simulink model "gerbang_logika"  (R2025a)
settings: Solver=VariableStepAuto  StartTime=0.0  StopTime=10.0  RelTol=1e-3
settings Model: Creator=pasha  LastModifiedBy=pasha

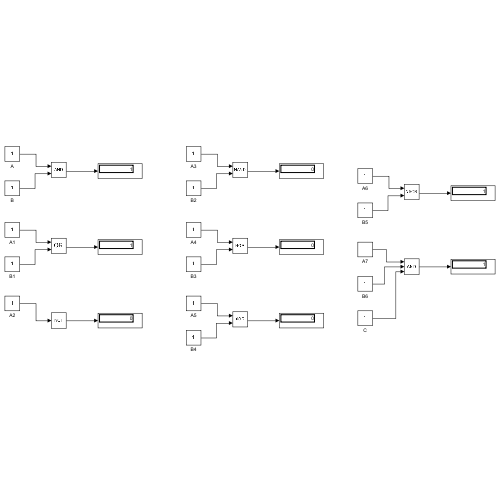
[thumbnail: Simulink's stored preview of the top-level diagram]
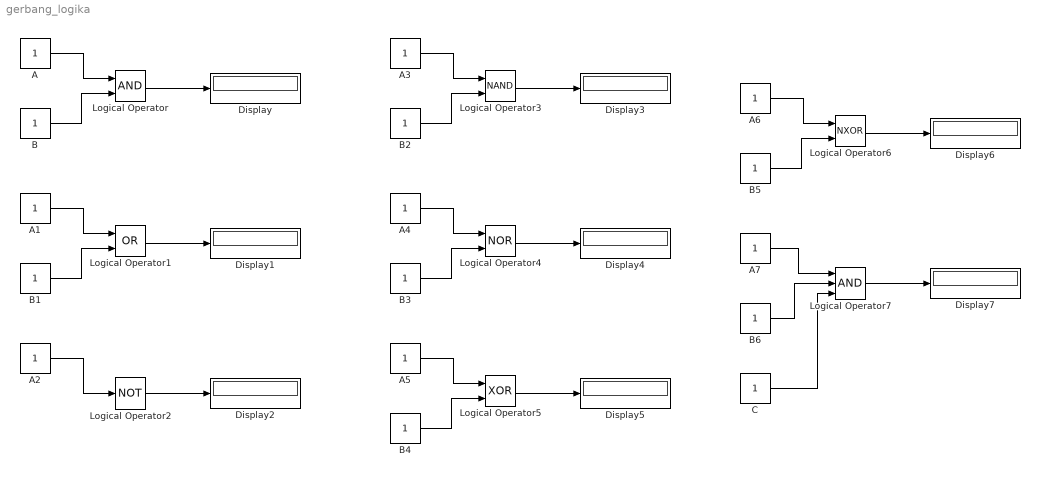
== system gerbang_logika ==
  A{,1..7} (8 alike) : Constant
  B{,1..6} (7 alike) : Constant
  C : Constant
  Display{,1..7} (8 alike) : Display
  Logical Operator : Logic  AllPortsSameDT=off  OutDataTypeStr=boolean
  Logical Operator1 : Logic  Operator=OR  AllPortsSameDT=off  OutDataTypeStr=boolean
  Logical Operator2 : Logic  Operator=NOT  AllPortsSameDT=off  OutDataTypeStr=boolean
  Logical Operator3 : Logic  Operator=NAND  AllPortsSameDT=off  OutDataTypeStr=boolean
  Logical Operator4 : Logic  Operator=NOR  AllPortsSameDT=off  OutDataTypeStr=boolean
  Logical Operator5 : Logic  Operator=XOR  AllPortsSameDT=off  OutDataTypeStr=boolean
  Logical Operator6 : Logic  Operator=NXOR  AllPortsSameDT=off  OutDataTypeStr=boolean
  Logical Operator7 : Logic  Inputs=3  AllPortsSameDT=off  OutDataTypeStr=boolean
  wires:
  A/1 -> Logical Operator/1
  B/1 -> Logical Operator/2
  Logical Operator/1 -> Display/1
  B1/1 -> Logical Operator1/2
  Logical Operator1/1 -> Display1/1
  A1/1 -> Logical Operator1/1
  A2/1 -> Logical Operator2/1
  Logical Operator2/1 -> Display2/1
  B2/1 -> Logical Operator3/2
  Logical Operator3/1 -> Display3/1
  A3/1 -> Logical Operator3/1
  Logical Operator4/1 -> Display4/1
  B3/1 -> Logical Operator4/2
  A4/1 -> Logical Operator4/1
  A5/1 -> Logical Operator5/1
  B4/1 -> Logical Operator5/2
  Logical Operator5/1 -> Display5/1
  A6/1 -> Logical Operator6/1
  B5/1 -> Logical Operator6/2
  Logical Operator6/1 -> Display6/1
  B6/1 -> Logical Operator7/2
  A7/1 -> Logical Operator7/1
  Logical Operator7/1 -> Display7/1
  C/1 -> Logical Operator7/3
